simulink model "pendulo_resorte"  (R2018a)
settings: Solver=FixedStepAuto  StartTime=0.0  StopTime=10  FixedStep=1e-3  MaxStep=1e-3  RelTol=1e-3
libraries: simulink x3
settings Model: Creator=carma  LastModifiedBy=carma

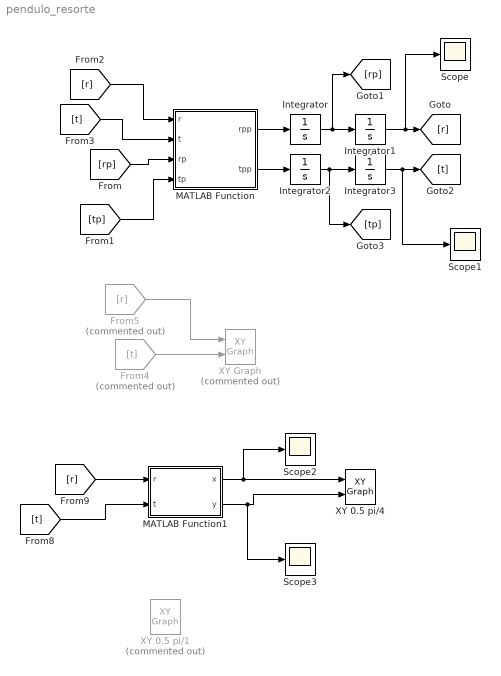
== system pendulo_resorte ==
  From4 : From  Commented=on  GotoTag=t
  From5 : From  Commented=on  GotoTag=r
  Integrator : Integrator
  Integrator1 : Integrator  InitialCondition=0.5
  Integrator2 : Integrator
  Integrator3 : Integrator  InitialCondition=pi/8
  MATLAB Function : MATLAB Function  TreatAsAtomicUnit=on
  MATLAB Function1 : MATLAB Function  TreatAsAtomicUnit=on
  Scope{,1..3} (4 alike) : Scope
  XY 0.5 pi/1 : simulink/Sinks/XY Graph  Commented=on  xmin=-0.15  xmax=0.15  ymin=-0.55  ymax=-0.49  st=-1
  XY 0.5 pi/4 : simulink/Sinks/XY Graph  xmin=-0.5  xmax=0.45  ymin=-0.75  ymax=-0.35  st=-1
  XY Graph : simulink/Sinks/XY Graph  Commented=on  xmin=0.5  xmax=0.75  ymin=-0.82  ymax=0.82  st=-1
  wires:
  MATLAB Function/1(rpp) -> Integrator/1
  Integrator/1 -> [rp], Integrator1/1
  Integrator2/1 -> [tp], Integrator3/1
  MATLAB Function/2(tpp) -> Integrator2/1
  Integrator1/1 -> Scope/1, [r]
  Integrator3/1 -> Scope1/1, [t]
  [rp] -> MATLAB Function/3(rp)
  [tp] -> MATLAB Function/4(tp)
  [r] -> MATLAB Function/1(r)
  [t] -> MATLAB Function/2(t)
  From5/1 -> XY Graph/1
  From4/1 -> XY Graph/2
  [r] -> MATLAB Function1/1(r)
  [t] -> MATLAB Function1/2(t)
  MATLAB Function1/1(x) -> Scope2/1, XY 0.5 pi/4/1
  MATLAB Function1/2(y) -> Scope3/1, XY 0.5 pi/4/2

== matlab function pendulo_resorte/MATLAB Function1 ==
  data: x output; r input; y output; t input
function [x,y] = fcn(r,t)

x = r*sin(t);
y=-r*cos(t);

== matlab function pendulo_resorte/MATLAB Function ==
  data: r input; rpp output; t input; tpp output; rp input; tp input
function [rpp,tpp] = fcn(r,t,rp,tp)

%Parametros tsim=5
l=0.5;
m=1; %0.25
g=9.8;
k=100;

%caos tini=pi/8; tini=pi/4 no tan caotico

%Parametros caos tsim=50
% l=0.5;
% m=1; 
% g=9.8;
% k=100;
%ecuaciones

rpp=r*tp^2-(k/m)*(r-l)+g*cos(t);
tpp=-(2*rp*tp+g*sin(t))/r;
